simulink model "base_open_loop_model_compare4"  (R2017a)
settings: Solver=ode45  StartTime=0.0  StopTime=5  FixedStep=0.01  RelTol=1e-3  EnableMultiTasking=on
settings Model: Creator=cpmcclel  LastModifiedBy=s6bae
settings DataIOCC: LimitDataPoints=on  SaveFormat=Array
settings OptimizationCC: LifeSpan=inf
settings DebuggingCC: SolverPrmCheckMsg=warning  SFUnexpectedBacktrackingDiag=warning  SFNoUnconditionalDefaultTransitionDiag=warning  SFExecutionAtInitializationDiag=none
settings HardwareCC: ProdBitPerPointer=32  ProdBitPerSizeT=32  ProdBitPerPtrDiffT=32  ProdLargestAtomicFloat=None  ProdIntDivRoundTo=Undefined  ProdEndianess=Unspecified  ProdWordSize=32  ProdHWDeviceType=32-bit Generic
settings ModelReferenceCC: PropagateSignalLabelsOutOfModel=off
settings GRTTargetCC: TargetLangStandard=C89/C90 (ANSI)  GeneratePreprocessorConditionals=Disable all
settings ConfigComp: CovMetricSettings=dw  CovHtmlReporting=on  CovSaveCumulativeToWorkspaceVar=on  CovSaveSingleToWorkspaceVar=on  CovExternalEMLEnable=off  CovSFcnEnable=off

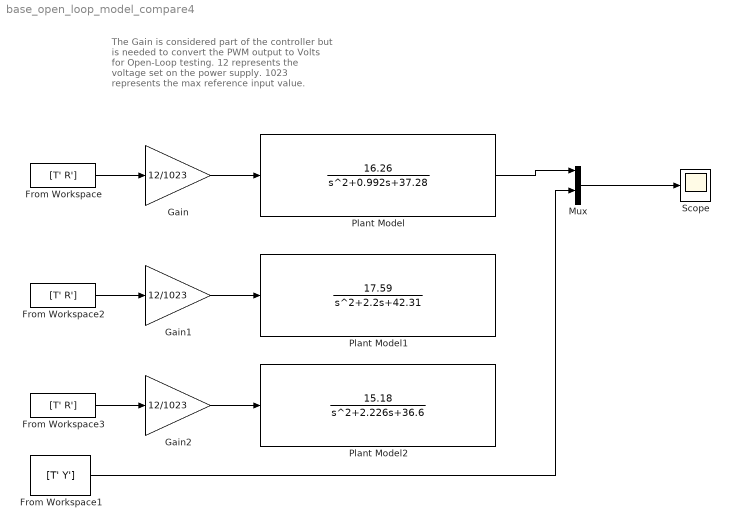
== system base_open_loop_model_compare4 ==
  note: The Gain is considered part of the controller but is needed to convert the PWM output to Volts for Open-Loop testing. 12 represents the voltage set on the power supply. 1023 represents the max reference input value.
  From Workspace : FromWorkspace  VariableName=[T' R']  SampleTime=.01
  From Workspace1 : FromWorkspace  VariableName=[T' Y']
  From Workspace2 : FromWorkspace  VariableName=[T' R']  SampleTime=.01
  From Workspace3 : FromWorkspace  VariableName=[T' R']  SampleTime=.01
  Gain : Gain  Gain=12/1023
  Gain1 : Gain  Gain=12/1023
  Gain2 : Gain  Gain=12/1023
  Mux : Mux
  Plant Model : TransferFcn  Numerator=[16.26]  Denominator=[1 0.992 37.28]
  Plant Model1 : TransferFcn  Numerator=[17.59]  Denominator=[1 2.2 42.31]
  Plant Model2 : TransferFcn  Numerator=[15.18]  Denominator=[1 2.226 36.6]
  Scope : Scope
  wires:
  From Workspace/1 -> Gain/1
  Mux/1 -> Scope/1
  From Workspace1/1 -> Mux/3
  Plant Model/1 -> Mux/1
  Gain/1 -> Plant Model/1
  From Workspace2/1 -> Gain1/1
  Gain1/1 -> Plant Model1/1
  From Workspace3/1 -> Gain2/1
  Gain2/1 -> Plant Model2/1
